simulink model "testFrame_ADCRawToIab"  (R2022b)
settings: Solver=FixedStepDiscrete  StartTime=0.0  StopTime=10.0  FixedStep=5e-05  RelTol=1e-3
libraries: simulink x2, SignalEditorBlockLib x1
settings Model: Creator=unix  LastModifiedBy=unix
settings SolverCC: AlgebraicLoopSolver=TrustRegion
settings DebuggingCC: UnconnectedInputMsg=warning  UnconnectedOutputMsg=warning  UnconnectedLineMsg=warning  SFMachineParentedDataDiag=warning
settings ModelReferenceCC: EnableRefExpFcnMdlSchedulingChecks=on
settings RTWCC: DLArmComputeVersion=19.05

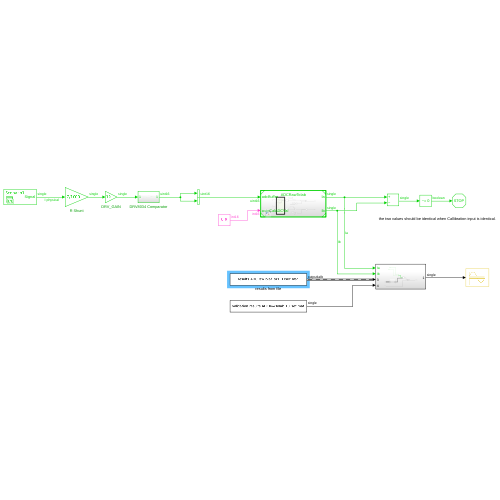
[thumbnail: Simulink's stored preview of the top-level diagram]
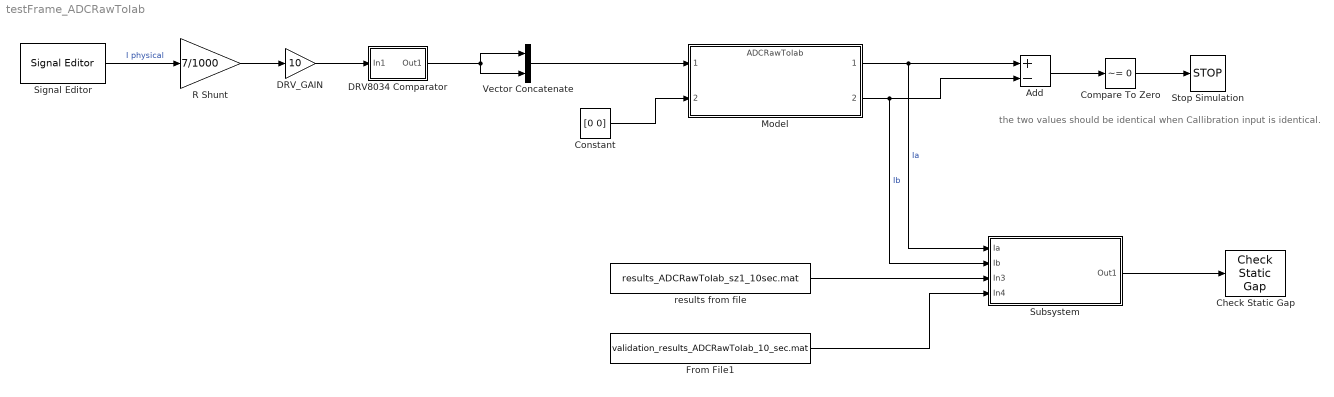
== system testFrame_ADCRawToIab ==
  note: the two values should be identical when Callibration input is identical.
  Add : Sum  Inputs=+-
  Check Static Gap : simulink/Model Verification/Check  Static Gap  Description=u <= -0.1 || 0 <= u  max=0  max_included=on  min=-0.1  min_included=on  enabled=on  stopWhenAssertionFail=on  export=off  icon=graphic
  Compare To Zero : simulink/Logic and Bit Operations/Compare To Zero  relop=~=  OutDataTypeStr=boolean
  Constant : Constant  Value=[0 0]  OutDataTypeStr=int16
  DRV8034 Comparator : Subsystem
  DRV_GAIN : Gain  Gain=10
  From File1 : FromFile  FileName=validation_results_ADCRawToIab_10_sec.mat  SampleTime=0
  Model : ModelReference  ModelNameDialog=ADCRawToIab.slx  SimulationMode=Accelerator  CachedPortDiscreteRates=[0.0002]  ModelReferenceVersion=7.2
  R Shunt : Gain  Gain=7/1000
  Signal Editor : SignalEditorBlockLib/Signal Editor  FileName=current_input_-30to30Amp.mat  ActiveScenario=Scenario1  ActiveSignal=Signal  IsBus=off  OutputBusObjectStr=Bus: BusObject  SampleTime=-1  Interpolate=off  ZeroCross=off  OutputAfterFinalValue=Setting to zero  Unit=inherit  PreserveSignalName=on
  Stop Simulation : Stop
  Subsystem : Subsystem
  Vector Concatenate : Concatenate
  results from file : FromFile  FileName=results_ADCRawToIab_sz1_10sec.mat  OutDataTypeStr=Bus: outputIaIb  SampleTime=0
  wires:
  Vector Concatenate/1 -> Model/1
  Model/1 -> Subsystem/1(Ia), Add/1  "Ia"
  Model/2 -> Subsystem/2(Ib), Add/2  "Ib"
  Signal Editor/1 -> R Shunt/1  "I physical"
  R Shunt/1 -> DRV_GAIN/1
  DRV_GAIN/1 -> DRV8034 Comparator/1(In1)
  DRV8034 Comparator/1(Out1) -> Vector Concatenate/2, Vector Concatenate/1
  Constant/1 -> Model/2
  Add/1 -> Compare To Zero/1
  Compare To Zero/1 -> Stop Simulation/1
  results from file/1 -> Subsystem/3(In3)
  From File1/1 -> Subsystem/4(In4)
  Subsystem/1(Out1) -> Check Static Gap/1

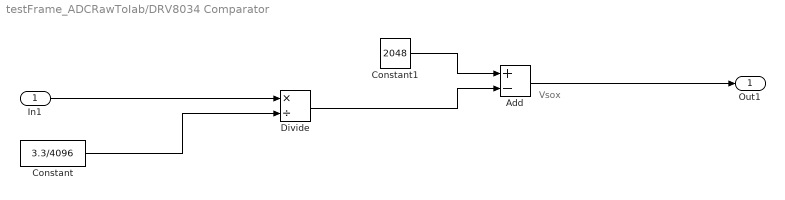
== system testFrame_ADCRawToIab/DRV8034 Comparator ==
  note: Vsox
  In1 : Inport
  Add : Sum  Inputs=+-  OutDataTypeStr=uint16  SaturateOnIntegerOverflow=on
  Constant : Constant  Value=3.3/4096
  Constant1 : Constant  Value=2048  OutDataTypeStr=uint16
  Divide : Product  Inputs=*/  OutDataTypeStr=int16
  Out1 : Outport
  wires:
  Constant/1 -> Divide/2
  Divide/1 -> Add/2
  Constant1/1 -> Add/1
  In1/1 -> Divide/1
  Add/1 -> Out1/1

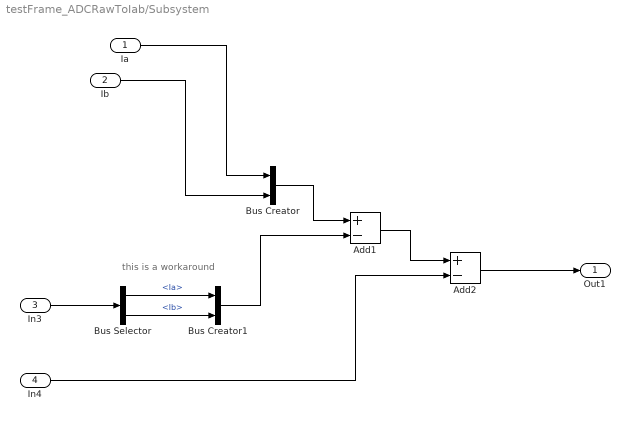
== system testFrame_ADCRawToIab/Subsystem ==
  note: this is a workaround
  Ia : Inport
  Ib : Inport  Port=2
  In3 : Inport  Port=3
  In4 : Inport  Port=4
  Add1 : Sum  Inputs=+-
  Add2 : Sum  Inputs=+-
  Bus Creator : BusCreator  Inputs=2  OutDataTypeStr=Bus: outputIaIb
  Bus Creator1 : BusCreator  Inputs=2
  Bus Selector : BusSelector  OutputSignals=Ia,Ib
  Out1 : Outport
  wires:
  Bus Selector/2 -> Bus Creator1/2  "<Ib>"
  Add1/1 -> Add2/1
  Bus Selector/1 -> Bus Creator1/1  "<Ia>"
  Bus Creator1/1 -> Add1/2
  Ia/1 -> Bus Creator/1
  Add2/1 -> Out1/1
  In4/1 -> Add2/2
  Bus Creator/1 -> Add1/1
  In3/1 -> Bus Selector/1
  Ib/1 -> Bus Creator/2
